simulink library "DAEMOT_Lib"  (R2019b)
settings: Solver=ode45  StartTime=0.0  StopTime=10.0  FixedStep=0.1  RelTol=1e-3
undefined symbols (not defined in the file or in its folder): Controller, CP, Ctrl, Ctrl_Fcn, Elec1, f, F2, Fluid, lag1, Mission, Moody, PropellerProp, rev_comms_sink
libraries: $bdroot x200, instrumentlib x21, simulink x5, dspsigops x2
(part 10 of 13)

== system DAEMOT_Lib/Support Functions/Real-Time Communication ==
  note: These blocks can be used to debug a controller that you want to run on hardware. With these blocks, the controller can be verified with a simulated plant. When transitioning to the hardware, simply replace these blocks with the non-debug version. At some point, it may be useful to combine the debug and non-debug versions into a single block. Maybe a task best saved for a rainy day :)
  note: We might be able to merge these two. I was never able to figure out if a combined block affected the output? However, the split format may be better for debugging purposes...
  LabVIEW_UDP : Subsystem  mask(LabView Measurements){n_in=[], n_out=[], config_loc=C:\Users\aksland2\BoxS\Box Sync\Research\Graduate Research\Models\UDP Communications Blocks\Matlab.json}
      mask prompts: n_in "Number of measurements from LabView"; n_out "Number of measurements to LabView"; config_loc "LabVIEW Config File Location (.json)"
      mask help: This block sends data to and from LabVIEW over UDP. The bus names are taken from a configuration file generated within LabVIEW. The update rate is hard-coded to 10 Hz.
      mask init:
      | h      = get_param(gcb,'handle');   % Get block handle
      | blk    = gcb;
      | hblock = get(h);     % Parse out handles structure
      | 
      | % Load .json file
      | fname = config_loc;
      | fid = fopen(fname);
      | raw = fread(fid,inf);
      | str = char(raw');
      | fclose(fid);
      | val = jsondecode(str);
      | 
      | % Retrieve data of interest
      | signals_in = val{1,1};
      | signals_out = val{2,1};
      | 
      | % Remove empty cells
      | signals_in  = signals_in(~cellfun(@isempty,signals_in));
      | signals_out = signals_out(~cellfun(@isempty,signals_out));
      | 
      | n_in  = length(signals_in);
      | n_out = length(signals_out);
      | 
      | % Set Demux and Bus Creator dimensions
      | set_param([blk,'/Demux'],'Outputs',num2str(n_in));
      | set_param([blk,'/Bus Creator'],'Inputs',num2str(n_in));
      | set_param([blk,'/UDP Receive/'],'DataSize',['[', num2str(n_in), ' 1]']);
      | 
      | % Get line handles
      | p = get_param([blk,'/Demux'],'PortHandles');
      | % l = get_param(p.Outport,'Line');
      | 
      | for i=1:n_in
      |     try
      |         % Draw lines
      |         add_line(blk,['Demux/',num2str(i)], ['Bus Creator/',num2str(i)],'AutoRouting','on')
      |     catch
      |         set_param(p.Outport(i),'Name',signals_in{i})
      |     end
      | end
      | 
      | delete_unconnected_lines(blk);
      | 
      | % Generate string of bus names to LabVIEW
      | out_str = '';
      | for i=1:n_out-1
      |     out_str = [out_str,[signals_out{i},',']];
      | end
      | out_str = [out_str,signals_out{n_out}];
      | 
      | set_param([blk,'/Bus Selector'],'OutputSignals',out_str);
      mask Display:
      | port_label('input',1,['Bus to LabVIEW - ',num2str(n_out),' signals'])
      | port_label('output',1,['Bus from LabVIEW - ',num2str(n_in),' signals'])
  UDP_Controller : Subsystem  Priority=2  mask{ctrl_fcn=[1*u(1)], conn=1, update_rate=.1, send_rate=Ctrl.dtSend, in_size=10, out_size=10, port_in=61177, loc_port_in=61176, port_out=61167, loc_port_out=61166}
      mask prompts: ctrl_fcn "Controller Function Name"; conn "Connection Number [1-10]"; update_rate "Controller Update Rate (s)"; send_rate "Send Rate [s]"; in_size "Controller Input Size"; out_size "Controller Output Size"; port_in "Input Port"; loc_port_in "Input Local Port"; port_out "Output Port"; loc_port_out "Output Local Port"
      mask help: Solves a controller with inputs/outputs sent over a UDP connection. The UDP Receive sample time is set to the controller update rate.
      mask init:
      | block = gcb;
      | 
      | port_in     = '61577';
      | loc_port_in = '61576';
      | 
      | port_out     = '61567';
      | loc_port_out = '61566';
      | 
      | port_in      = [port_in(1:2)     ,conn,port_in(4:5)];
      | loc_port_in  = [loc_port_in(1:2) ,conn,loc_port_in(4:5)];
      | port_out     = [port_out(1:2)    ,conn,port_out(4:5)];
      | loc_port_out = [loc_port_out(1:2),conn,loc_port_out(4:5)];
      | 
      | set_param(gcb,'port_in'     ,port_in);
      | set_param(gcb,'loc_port_in' ,loc_port_in);
      | set_param(gcb,'port_out'    ,port_out);
      | set_param(gcb,'loc_port_out',loc_port_out);
      | 
      | set_param([gcb,'/Controller/Controller'],'MATLABFcn',ctrl_fcn);
      | set_param([gcb,'/Controller/Controller'],'OutputDimensions',num2str(out_size));
      | set_param([gcb,'/Controller'],'SystemSampleTime',num2str(update_rate));
      | 
      | set_param([gcb,'/UDP Receive'],'Port',port_in);
      | set_param([gcb,'/UDP Receive'],'LocalPort',loc_port_in);
      | set_param([gcb,'/UDP Receive'],'SampleTime',num2str(update_rate));
      | set_param([gcb,'/UDP Receive'],'Timeout',num2str(update_rate+5));
      | set_param([gcb,'/UDP Receive'],'DataSize',['[', num2str(in_size), ' 1]']);
      | 
      | 
      | 
      | % set_param([gcb,'/From Controller'],'SystemSampleTime',num2str(update_rate));
      | set_param([gcb,'/From Controller/UDP Send'],'Port',port_out);
      | set_param([gcb,'/From Controller/UDP Send'],'LocalPort',loc_port_out);
      | set_param([gcb,'/From Controller'],'SystemSampleTime',num2str(update_rate));
      | 
      | set_param(bdroot,'FixedStep',num2str(update_rate))
      mask Display:
      | disp(['UDP Controller\n\nFunction: ',ctrl_fcn,'\n\nConnection: ',conn,'\n\nUpdate Rate (s): ',num2str(update_rate),'s\n\nInput Size: ',num2str(in_size),'\n\nOutput Size: ',num2str(out_size)])
      | 
      | % disp(['UDP Controller\n\nFunction: ',ctrl_fcn,'\n\nConnection: ',conn,'\n\nUpdate Rate (s): ',num2str(update_rate),'\n\nSend Rate (s): ',num2str(send_rate),'s\n\nInput Size: ',num2str(in_size),'\n\nOutput Size: ',num2str(out_size)])
  UDP_Controller_Debug : Subsystem  Priority=2  AncestorBlock=DAEMOT_Lib_2016a/Support Functions/UDP_Controller  mask{ctrl_fcn=Controller(u), conn=1, update_rate=.1, send_rate=.1, in_size=10, out_size=10, port_in=61177, loc_port_in=61176, port_out=61167, loc_port_out=61166}
      mask prompts: ctrl_fcn "Controller Function Name"; conn "Connection Number [1-10]"; update_rate "Controller Update Rate (s)"; send_rate "Send Rate [s]"; in_size "Controller Input Size"; out_size "Controller Output Size"; port_in "Input Port"; loc_port_in "Input Local Port"; port_out "Output Port"; loc_port_out "Output Local Port"
      mask help: Solves a controller with inputs/outputs sent over a UDP connection. The UDP Receive sample time is set to the controller update rate.
      mask init:
      | block = gcb;
      | 
      | port_in     = '61577';
      | loc_port_in = '61576';
      | 
      | port_out     = '61567';
      | loc_port_out = '61566';
      | 
      | port_in      = [port_in(1:2)     ,conn,port_in(4:5)];
      | loc_port_in  = [loc_port_in(1:2) ,conn,loc_port_in(4:5)];
      | port_out     = [port_out(1:2)    ,conn,port_out(4:5)];
      | loc_port_out = [loc_port_out(1:2),conn,loc_port_out(4:5)];
      | 
      | set_param(gcb,'port_in'     ,port_in);
      | set_param(gcb,'loc_port_in' ,loc_port_in);
      | set_param(gcb,'port_out'    ,port_out);
      | set_param(gcb,'loc_port_out',loc_port_out);
      | 
      | set_param([gcb,'/Controller'],'MATLABFcn',ctrl_fcn);
      | set_param([gcb,'/Controller'],'OutputDimensions',num2str(out_size));
      | 
      | set_param([gcb,'/UDP Receive'],'Port',port_in);
      | set_param([gcb,'/UDP Receive'],'LocalPort',loc_port_in);
      | set_param([gcb,'/UDP Receive'],'SampleTime',num2str(update_rate));
      | set_param([gcb,'/UDP Receive'],'Timeout',num2str(update_rate+5));
      | set_param([gcb,'/UDP Receive'],'DataSize',['[', num2str(in_size), ' 1]']);
      | 
      | 
      | 
      | % set_param([gcb,'/From Controller'],'SystemSampleTime',num2str(update_rate));
      | set_param([gcb,'/From Controller/UDP Send'],'Port',port_out);
      | set_param([gcb,'/From Controller/UDP Send'],'LocalPort',loc_port_out);
      | set_param([gcb,'/From Controller'],'SystemSampleTime',num2str(send_rate));
      | 
      | set_param(bdroot,'FixedStep',num2str(update_rate))
      mask Display: disp(['UDP Controller\n\nFunction: ',ctrl_fcn,'\n\nConnection: ',conn,'\n\nUpdate Rate (s): ',num2str(update_rate),'\n\nSend Rate (s): ',num2str(send_rate),'s\n\nInput Size: ',num2str(in_size),'\n\nOutput Size: ',num2str(out_size)])
  UDP_Controller_Recieve : Subsystem  mask(Send/Receive to UDP Controller){conn=1, update_rate=.1, rec_rate=.1, out_size=10, Initial=zeros(10,1), port_out=61166, loc_port_out=61167}
      mask prompts: conn "Connection Number [1-10]"; update_rate "Controller Update Rate (s)"; rec_rate "Recieve Rate [s]"; out_size "Controller Output Size"; Initial "Initial Output"; port_out "Output Port"; loc_port_out "Output Local Port"
      mask help: Sends and retrieves data from a controller over a UDP connection. Passes data over UDP at 10 Hz but applies a sample and hold at the update rate of the controller.
      mask init:
      | block = gcb;
      | 
      | % port_in     = '61576';
      | % loc_port_in = '61577';
      | 
      | port_out     = '61566';
      | loc_port_out = '61567';
      | 
      | % port_in      = [port_in(1:2)     ,conn,port_in(4:5)];
      | % loc_port_in  = [loc_port_in(1:2) ,conn,loc_port_in(4:5)];
      | port_out     = [port_out(1:2)    ,conn,port_out(4:5)];
      | loc_port_out = [loc_port_out(1:2),conn,loc_port_out(4:5)];
      | % 
      | % set_param(gcb,'port_in'     ,port_in);
      | % set_param(gcb,'loc_port_in' ,loc_port_in);
      | set_param(gcb,'port_out'    ,port_out);
      | set_param(gcb,'loc_port_out',loc_port_out);
      | % 
      | % set_param([gcb,'/To Controller/UDP Send'],'Port',port_in);
      | % set_param([gcb,'/To Controller/UDP Send'],'LocalPort',loc_port_in);
      | 
      | % test2 = ['[', num2str(out_size), ' 1]']
      | set_param([gcb,'/UDP Receive'],'Port',port_out);
      | set_param([gcb,'/UDP Receive'],'LocalPort',loc_port_out);
      | set_param([gcb,'/UDP Receive'],'DataSize',['[', num2str(out_size), ' 1]']);
      | set_param([gcb,'/UDP Receive'],'SampleTime',num2str(rec_rate));
      | 
      | set_param([gcb,'/Zero-Order Hold'],'SampleTime',num2str(update_rate));
      mask Display: disp(['Receive from UDP Controller\n\nConnection: ',conn,'\n\nUpdate Rate (s): ',num2str(update_rate),'\n\nReceive Rate (s): ',num2str(rec_rate),'\n\nOutput Size: ',num2str(out_size)])
  UDP_Controller_Recieve_Debug : Subsystem  Priority=3  AncestorBlock=DAEMOT_Lib_2016a/Support Functions/UDP_Controller_SR  mask(Send/Receive to UDP Controller){conn=1, update_rate=10, rec_rate=.1, out_size=10, Initial=zeros(10,1), port_out=61166, loc_port_out=61167}
      mask prompts: conn "Connection Number [1-10]"; update_rate "Controller Update Rate (s)"; rec_rate "Recieve Rate [s]"; out_size "Controller Output Size"; Initial "Initial Output"; port_out "Output Port"; loc_port_out "Output Local Port"
      mask help: Sends and retrieves data from a controller over a UDP connection. Passes data over UDP at 10 Hz but applies a sample and hold at the update rate of the controller.
      mask init:
      | block = gcb;
      | 
      | % port_in     = '61576';
      | % loc_port_in = '61577';
      | 
      | port_out     = '61566';
      | loc_port_out = '61567';
      | 
      | % port_in      = [port_in(1:2)     ,conn,port_in(4:5)];
      | % loc_port_in  = [loc_port_in(1:2) ,conn,loc_port_in(4:5)];
      | port_out     = [port_out(1:2)    ,conn,port_out(4:5)];
      | loc_port_out = [loc_port_out(1:2),conn,loc_port_out(4:5)];
      | % 
      | % set_param(gcb,'port_in'     ,port_in);
      | % set_param(gcb,'loc_port_in' ,loc_port_in);
      | set_param(gcb,'port_out'    ,port_out);
      | set_param(gcb,'loc_port_out',loc_port_out);
      | % 
      | % set_param([gcb,'/To Controller/UDP Send'],'Port',port_in);
      | % set_param([gcb,'/To Controller/UDP Send'],'LocalPort',loc_port_in);
      | 
      | % test2 = ['[', num2str(out_size), ' 1]']
      | set_param([gcb,'/UDP Receive'],'Port',port_out);
      | set_param([gcb,'/UDP Receive'],'LocalPort',loc_port_out);
      | set_param([gcb,'/UDP Receive'],'DataSize',['[', num2str(out_size), ' 1]']);
      | set_param([gcb,'/UDP Receive'],'SampleTime',num2str(rec_rate));
      mask Display: disp(['Receive from UDP Controller\n\nConnection: ',conn,'\n\nUpdate Rate (s): ',num2str(update_rate),'\n\nReceive Rate (s): ',num2str(rec_rate),'\n\nOutput Size: ',num2str(out_size)])
  UDP_Controller_Send : Subsystem  mask(Send/Receive to UDP Controller){conn=1, update_rate=.1, in_size=10, port_in=61176, loc_port_in=61177}
      mask prompts: conn "Connection Number [1-10]"; update_rate "Controller Update Rate (s)"; in_size "Controller Input Size"; port_in "Input Port"; loc_port_in "Input Local Port"
      mask help: Sends and retrieves data from a controller over a UDP connection. Passes data over UDP at 10 Hz but applies a sample and hold at the update rate of the controller.
      mask init:
      | block = gcb;
      | 
      | port_in     = '61576';
      | loc_port_in = '61577';
      | 
      | % port_out     = '61566';
      | % loc_port_out = '61567';
      | 
      | port_in      = [port_in(1:2)     ,conn,port_in(4:5)];
      | loc_port_in  = [loc_port_in(1:2) ,conn,loc_port_in(4:5)];
      | % port_out     = [port_out(1:2)    ,conn,port_out(4:5)];
      | % loc_port_out = [loc_port_out(1:2),conn,loc_port_out(4:5)];
      | 
      | set_param(gcb,'port_in'     ,port_in);
      | set_param(gcb,'loc_port_in' ,loc_port_in);
      | % set_param(gcb,'port_out'    ,port_out);
      | % set_param(gcb,'loc_port_out',loc_port_out);
      | 
      | set_param([gcb,'/To Controller/UDP Send'],'Port',port_in);
      | set_param([gcb,'/To Controller/UDP Send'],'LocalPort',loc_port_in);
      | set_param([gcb,'/To Controller'],'SystemSampleTime',num2str(update_rate));
      | 
      | % set_param([gcb,'/From Controller/MEASUREMENTS1/UDP Receive'],'Port',port_out);
      | % set_param([gcb,'/From Controller/MEASUREMENTS1/UDP Receive'],'LocalPort',loc_port_out);
      mask Display:
      | disp(['Send to UDP Controller\n\nConnection: ',conn,'\n\nUpdate Rate (s): ',num2str(update_rate),'s\n\nInput Size: ',num2str(in_size)])
      | % disp(['Send/Receive to UDP Controller\n\nConnection: ',conn,'\n\nUpdate Rate (s): ',num2str(update_rate),'s\n\nInput Size: ',num2str(in_size),'\n\nOutput Size: ',num2str(out_size)])
  UDP_Controller_Send_Debug : Subsystem  Priority=1  AncestorBlock=DAEMOT_Lib_2016a/Support Functions/UDP_Controller_SR  mask(Send/Receive to UDP Controller){conn=1, update_rate=.1, in_size=10, port_in=61176, loc_port_in=61177}
      mask prompts: conn "Connection Number [1-10]"; update_rate "Controller Update Rate (s)"; in_size "Controller Input Size"; port_in "Input Port"; loc_port_in "Input Local Port"
      mask help: Sends and retrieves data from a controller over a UDP connection. Passes data over UDP at 10 Hz but applies a sample and hold at the update rate of the controller.
      mask init: same as DAEMOT_Lib/Support Functions/Real-Time Communication/UDP_Controller_Send
      mask Display:
      | disp(['Send to UDP Controller\n\nConnection: ',conn,'\n\nUpdate Rate (s): ',num2str(update_rate),'s\n\nInput Size: ',num2str(in_size)])
      | % disp(['Send/Receive to UDP Controller\n\nConnection: ',conn,'\n\nUpdate Rate (s): ',num2str(update_rate),'s\n\nInput Size: ',num2str(in_size),'\n\nOutput Size: ',num2str(out_size)])

== system DAEMOT_Lib/Support Functions/Sink ==
  In1 : Inport
  tag scope: gdata_DAEMOT_LibSupportFunctionsSink=global
  wires:
  In1/1 -> [gdata_DAEMOT_LibSupportFunctionsSink]

== system DAEMOT_Lib/Support Functions/Source ==
  Out1 : Outport  VectorParamsAs1DForOutWhenUnconnected=off
  wires:
  [gdata_Thermal_System_BUSM2FSink2] -> Out1/1

== system DAEMOT_Lib/Support Functions/Unit Conversion  ==
  Signal_in : Inport
  conv_fcn : Fcn  Expr=(u(1)+459.67)/1.8-273.15
  Converted Signal Out : Outport  VectorParamsAs1DForOutWhenUnconnected=off
  wires:
  conv_fcn/1 -> Converted Signal Out/1
  Signal_in/1 -> conv_fcn/1

== system DAEMOT_Lib/Support Functions/Upper to Lower Edge Preview ==
  Trajectory : Inport
  Digital Clock : DigitalClock  SampleTime=dt_u
  Mission Preview1 : Subsystem  TreatAsAtomicUnit=on  SystemSampleTime=dt_l
  Scope : Scope
  Reference : Outport
  wires:
  Mission Preview1/1(References) -> Reference/1, Scope/1
  Trajectory/1 -> Mission Preview1/1(Trajectory)
  Digital Clock/1 -> Mission Preview1/2(Time)

== system DAEMOT_Lib/Support Functions/Upper to Lower Mission Preview ==
  Current State : Inport
  Trajectory : Inport  Port=2
  Bias1 : Bias  Bias=dt_l*linspace(0,(hor_l-1),hor_l)+dt_l
  Constant : Constant  Value=opts
  Constant1 : Constant  Value=dt_u*linspace(1,hor_u,hor_u)
  Constant2 : Constant  Value=ones(hor_u,1)  SampleTime=-1
  Constant4 : Constant  Value=dt_u  SampleTime=-1
  Digital Clock1 : DigitalClock  SampleTime=dt_l
  Lookup Table Dynamic : simulink/Lookup Tables/Lookup Table Dynamic  LookUpMeth=Interpolation-Use End Values  OutDataType=fixdt('double')  OutScaling=[]  OutputDataTypeScalingMode=Specify via dialog  OutDataTypeStr=fixdt('double')  DoSatur=off
      settings: SourceProductName=Simulink
  Math Function : Math  Operator=mod  SaturateOnIntegerOverflow=on
  Mux1 : Mux  Inputs=2
  Mux2 : Mux  Inputs=2
  Product : Product
  Selector : Selector  InputPortWidth=hor_u  IndexOptions=Index vector (dialog)  Indices=1  OutputSizes=1
  Switch : Switch  Criteria=u2 > Threshold
  Reference : Outport  VectorParamsAs1DForOutWhenUnconnected=off
  wires:
  Constant4/1 -> Math Function/2
  Digital Clock1/1 -> Math Function/1
  Constant/1 -> Switch/2
  Switch/1 -> Mux1/2
  Current State/1 -> Mux1/1
  Trajectory/1 -> Selector/1, Switch/3
  Mux1/1 -> Lookup Table Dynamic/3
  Mux2/1 -> Lookup Table Dynamic/2
  Constant1/1 -> Mux2/2
  Math Function/1 -> Bias1/1, Mux2/1
  Bias1/1 -> Lookup Table Dynamic/1
  Lookup Table Dynamic/1 -> Reference/1
  Product/1 -> Switch/1
  Selector/1 -> Product/2
  Constant2/1 -> Product/1

== system DAEMOT_Lib/Thermal/Air Volume ==
  In1 : Inport
  In2 : Inport  Port=2
  Q : Inport  Port=3
  Air_Volume : MATLAB Function  TreatAsAtomicUnit=on
  Bus Creator2 : BusCreator  Inputs=3
  Bus Selector1 : BusSelector  OutputSignals=Q_kW,Temp
  Constant : Constant  Value=P_init
  Constant1 : Constant  Value=T_init
  Data_Sink1 : $bdroot/Support Functions/Data_Sink
  Demux : Demux  Outputs=3
  Integrate : Integrator  InitialCondition=[T_init P_init M_init]  LimitOutput=on
  Sink1 : $bdroot/Support Functions/Sink
  Sink2 : $bdroot/Support Functions/Sink  Commented=on
  Source1 : $bdroot/Support Functions/Source
  Terminator : Terminator
  Terminator1 : Terminator
  b1 : BusCreator  Inputs=3
  gb1 : BusSelector  OutputSignals=mdot_kgps,T_C,P_kPa
  kW to W : Gain  Gain=1e3
  n-D Lookup Table1 : Lookup_n-D  BreakpointsForDimension1=Fluid.P  BreakpointsForDimension2=Fluid.T  BreakpointsForDimension3=[5, 7]  Table=Fluid.C_pt  ExtrapMethod=Clip  UseLastTableValue=on  RndMeth=Simplest  InputSameDT=on
  n-D Lookup Table2 : Lookup_n-D  BreakpointsForDimension1=Fluid.P  BreakpointsForDimension2=Fluid.T  BreakpointsForDimension3=[5, 7]  Table=Fluid.Rho_pt  ExtrapMethod=Clip  UseLastTableValue=on  RndMeth=Simplest  InputSameDT=on
  pout1 : From  Commented=on  GotoTag=T_tank
  Out1 : Outport  VectorParamsAs1DForOutWhenUnconnected=off
  wires:
  b1/1 -> Out1/1
  [Mdot_out] -> b1/1  "mdot_kgps"
  gb1/2 -> [T_in]  "<T_C>"
  [T_tank] -> b1/2  "T_C"
  gb1/1 -> [Mdot_in]  "<mdot_kgps>"
  In1/1 -> gb1/1
  [P_tank] -> b1/3  "P_kPa"
  gb1/3 -> Terminator/1  "<P_kPa>"
  [P_tank] -> Sink1/1
  Source1/1 -> [Mdot_out]
  In2/1 -> [T_amb]
  [Mdot_in] -> Air_Volume/2(Mdot_in)
  [Mdot_out] -> Air_Volume/3(Mdot_out)
  Air_Volume/1(x_dot) -> Integrate/1
  Integrate/1 -> Air_Volume/1(x), Demux/1
  Demux/1 -> [T_tank]
  Demux/2 -> [P_tank]
  Constant1/1 -> n-D Lookup Table2/2, n-D Lookup Table1/2
  Constant/1 -> n-D Lookup Table2/1, n-D Lookup Table1/1
  n-D Lookup Table1/1 -> Air_Volume/6(Cp)
  n-D Lookup Table2/1 -> Air_Volume/7(Rho)
  [T_in] -> Air_Volume/4(T_in)
  [T_amb] -> Air_Volume/5(T_amb)
  Bus Creator2/1 -> Data_Sink1/1
  [T_tank] -> Bus Creator2/1  "T"
  [P_tank] -> Bus Creator2/2  "P"
  [M_tank] -> Bus Creator2/3  "M"
  kW to W/1 -> Air_Volume/8(Q)
  Demux/3 -> [M_tank]
  pout1/1 -> Sink2/1
  Bus Selector1/2 -> Terminator1/1  "<Temp>"
  Bus Selector1/1 -> kW to W/1  "<Q_kW>"
  Q/1 -> Bus Selector1/1

== system DAEMOT_Lib/Thermal/Cold_Plate ==
  In1 : Inport
  Q : Inport  Port=2
  Bus Creator2 : BusCreator  Inputs=7
  Bus Selector : BusSelector  OutputSignals=Q_kW,Temp
  Cold_Plate : MATLAB Function  TreatAsAtomicUnit=on
  Constant2 : Constant  Value=Fluid.Bulk_Mod
  Demux : Demux  Outputs=3
  Integrate : Integrator  InitialCondition=[T_init P_init Tw_init]
  Mdot : MATLAB Function  TreatAsAtomicUnit=on
  Sink1 : $bdroot/Support Functions/Sink
  Sink2 : $bdroot/Support Functions/Sink
  Source1 : $bdroot/Support Functions/Source
  Terminator : Terminator
  Terminator2 : Terminator
  b1 : BusCreator  Inputs=3
  data_sink1 : $bdroot/Support Functions/Data_Sink
  gb1 : BusSelector  OutputSignals=mdot_kgps,T_C,P_kPa
  n-D Lookup Table1 : Lookup_n-D  BreakpointsForDimension1=Fluid.P  BreakpointsForDimension2=Fluid.T  BreakpointsForDimension3=[5, 7]  Table=Fluid.C_pt  ExtrapMethod=Clip  UseLastTableValue=on  RndMeth=Simplest  InputSameDT=on
  n-D Lookup Table2 : Lookup_n-D  BreakpointsForDimension1=Fluid.P  BreakpointsForDimension2=Fluid.T  BreakpointsForDimension3=[5, 7]  Table=Fluid.Rho_pt  ExtrapMethod=Clip  UseLastTableValue=on  RndMeth=Simplest  InputSameDT=on
  n-D Lookup Table8 : Lookup_n-D  BreakpointsForDimension1=Fluid.P  BreakpointsForDimension2=Fluid.T  BreakpointsForDimension3=[5, 7]  Table=Fluid.K_pt  ExtrapMethod=Clip  UseLastTableValue=on  RndMeth=Simplest  InputSameDT=on
  n-D Lookup Table9 : Lookup_n-D  BreakpointsForDimension1=Fluid.P  BreakpointsForDimension2=Fluid.T  BreakpointsForDimension3=[5, 7]  Table=Fluid.Mu_pt  ExtrapMethod=Clip  UseLastTableValue=on  RndMeth=Simplest  InputSameDT=on
  Out1 : Outport  VectorParamsAs1DForOutWhenUnconnected=off
  wires:
  b1/1 -> Out1/1
  [Mdot_down] -> b1/1  "mdot_kgps"
  gb1/2 -> [T_in]  "<T_C>"
  [T_out] -> b1/2  "T_C"
  gb1/1 -> Terminator2/1  "<mdot_kgps>"
  In1/1 -> gb1/1
  [P_out] -> b1/3  "P_kPa"
  gb1/3 -> [P_in]  "<P_kPa>"
  [Mdot] -> Sink1/1
  [Q_Load] -> Cold_Plate/2(Q_load)
  Source1/1 -> [Mdot_down]
  [T_in] -> Cold_Plate/6(T_in)
  Cold_Plate/1(x_dot) -> Integrate/1
  Bus Creator2/1 -> data_sink1/1
  [T_wall] -> Bus Creator2/4  "T_wall"
  [T_out] -> Bus Creator2/3  "T_out"
  [P_out] -> Bus Creator2/2  "P_out"
  [Q_Load] -> Bus Creator2/5  "Q_load"
  [Mdot] -> Bus Creator2/1  "Mdot"
  Cold_Plate/2(H) -> [H]  "HTC (W/m^2K)"
  [H] -> Bus Creator2/6  "HTC"
  n-D Lookup Table8/1 -> Cold_Plate/8(k)
  n-D Lookup Table9/1 -> Cold_Plate/7(mu)
  [T_out] -> n-D Lookup Table2/2, n-D Lookup Table9/2, n-D Lookup Table1/2, n-D Lookup Table8/2
  Integrate/1 -> Cold_Plate/1(x), Demux/1
  n-D Lookup Table1/1 -> Cold_Plate/9(Cp)
  Constant2/1 -> Cold_Plate/11(E_fluid)
  [Mdot_down] -> Cold_Plate/4(Mdot_down)
  [P_in] -> Cold_Plate/3(P_in)
  n-D Lookup Table2/1 -> Mdot/3(Rho), Cold_Plate/10(Rho)
  Mdot/1(Mdot) -> [Mdot], Cold_Plate/5(Mdot)
  [P_in] -> Mdot/1(P_in)
  [P_out] -> Mdot/2(P_out)
  Demux/2 -> [P_out]
  Demux/1 -> [T_out]
  Demux/3 -> [T_wall]
  [P_out] -> n-D Lookup Table2/1, n-D Lookup Table1/1, n-D Lookup Table8/1, n-D Lookup Table9/1
  Cold_Plate/3(Re) -> [Re]  "Re"
  [Re] -> Bus Creator2/7  "Re"
  Q/1 -> Bus Selector/1
  Bus Selector/1 -> [Q_Load]  "<Q_kW>"
  [T_wall] -> Sink2/1
  Bus Selector/2 -> Terminator/1  "<Temp>"

== system DAEMOT_Lib/Thermal/Flow Split_Junction ==
  In1 : Inport
  Bus Creator2 : BusCreator  Inputs=2
  Constant5 : Constant  Value=Fluid.Bulk_Mod
  Demux : Demux  Outputs=2
  Dynamic_Flow_Split_Junction : MATLAB Function  TreatAsAtomicUnit=on
  Integrator1 : Integrator  InitialCondition=[T_init P_init]
  Mux_In_1 : Mux  Inputs=1
  Mux_In_2 : Mux  Inputs=1
  Mux_In_3 : Mux  Inputs=1
  Selector1 : Selector  InputPortWidth=1  IndexOptions=Index vector (dialog)  Indices=[1 ]  OutputSizes=1
  Selector2 : Selector  InputPortWidth=1  IndexOptions=Index vector (dialog)  Indices=[1 ]  OutputSizes=1
  Sink1 : $bdroot/Support Functions/Sink
  Source1 : Subsystem
      mask init:
      | n_src = gcb;
      | n_src = str2num(n_src(end));
      | 
      | rev_comms_source(n_src);
      mask Display: text(0.25,0.5,'Source')
  b1 : BusCreator  Inputs=3
  data_sink1 : $bdroot/Support Functions/Data_Sink
  gb1 : BusSelector  OutputSignals=mdot_kgps,T_C,P_kPa
  gp1 : Terminator
  n-D Lookup Table2 : Lookup_n-D  BreakpointsForDimension1=Fluid.P  BreakpointsForDimension2=Fluid.T  BreakpointsForDimension3=[5, 7]  Table=Fluid.Rho_pt  ExtrapMethod=Clip  UseLastTableValue=on  RndMeth=Simplest  InputSameDT=on
  Out1 : Outport  VectorParamsAs1DForOutWhenUnconnected=off
  wires:
  b1/1 -> Out1/1
  [M_out1] -> b1/1  "mdot_kgps"
  gb1/2 -> [T_in1]  "<T_C>"
  [T] -> b1/2  "T_C"
  gb1/1 -> [M_in1]  "<mdot_kgps>"
  Source1/1(Out1) -> [M_out1]
  In1/1 -> gb1/1
  [P] -> b1/3  "P_kPa"
  gb1/3 -> gp1/1  "<P_kPa>"
  Mux_In_3/1 -> Selector2/1
  Mux_In_1/1 -> Selector1/1
  Mux_In_2/1 -> Dynamic_Flow_Split_Junction/3(Mdot_out)
  [M_in1] -> Mux_In_1/1
  [M_out1] -> Mux_In_2/1
  [T_in1] -> Mux_In_3/1
  [P] -> Sink1/1
  Dynamic_Flow_Split_Junction/1(x_dot) -> Integrator1/1
  Bus Creator2/1 -> data_sink1/1
  [T] -> Bus Creator2/1  "T_out"
  [P] -> Bus Creator2/2  "P"
  Integrator1/1 -> Demux/1, Dynamic_Flow_Split_Junction/1(x)
  Selector1/1 -> Dynamic_Flow_Split_Junction/2(Mdot_in)
  Constant5/1 -> Dynamic_Flow_Split_Junction/6(E_fluid)
  n-D Lookup Table2/1 -> Dynamic_Flow_Split_Junction/5(rho)
  [P] -> n-D Lookup Table2/1
  [T] -> n-D Lookup Table2/2
  Demux/1 -> [T]
  Demux/2 -> [P]
  Selector2/1 -> Dynamic_Flow_Split_Junction/4(T_in)

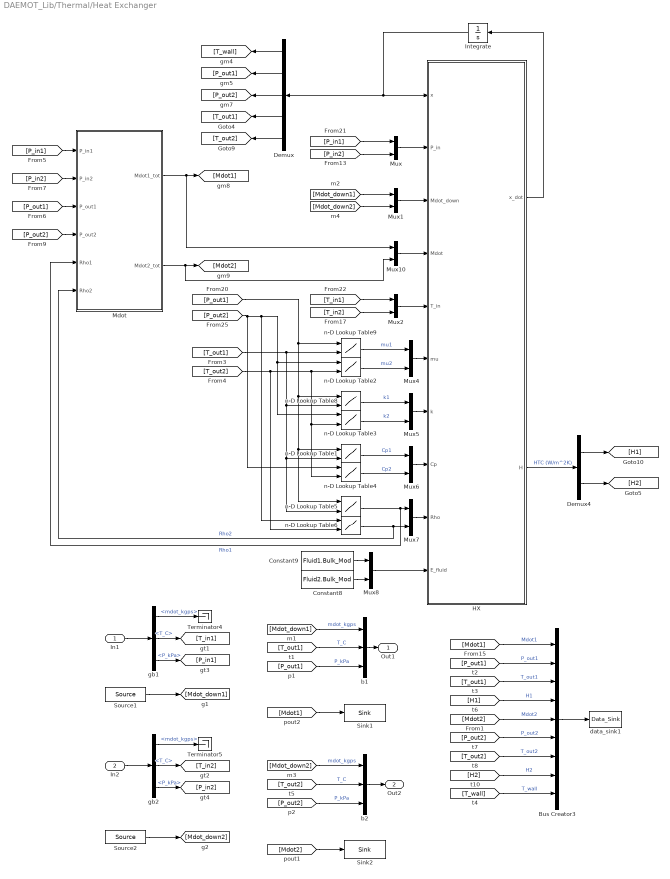
== system DAEMOT_Lib/Thermal/Heat Exchanger ==
  In1 : Inport
  In2 : Inport  Port=2
  Bus Creator3 : BusCreator  Inputs=9
  Constant8 : Constant  Value=Fluid2.Bulk_Mod
  Constant9 : Constant  Value=Fluid1.Bulk_Mod
  Demux : Demux  Outputs=5
  Demux4 : Demux  Outputs=2
  HX : MATLAB Function  TreatAsAtomicUnit=on
  Integrate : Integrator  InitialCondition=[Tw_init P1_init P2_init T1_init T2_init]
  Mdot : MATLAB Function  TreatAsAtomicUnit=on
  Mux{,1..2,4..8,10} (9 alike) : Mux  Inputs=2
  Sink1 : $bdroot/Support Functions/Sink
  Sink2 : $bdroot/Support Functions/Sink
  Source1 : $bdroot/Support Functions/Source
  Source2 : $bdroot/Support Functions/Source
  Terminator4 : Terminator
  Terminator5 : Terminator
  b1 : BusCreator  Inputs=3
  b2 : BusCreator  Inputs=3
  data_sink1 : $bdroot/Support Functions/Data_Sink
  gb1 : BusSelector  OutputSignals=mdot_kgps,T_C,P_kPa
  gb2 : BusSelector  OutputSignals=mdot_kgps,T_C,P_kPa
  n-D Lookup Table1 : Lookup_n-D  BreakpointsForDimension1=Fluid1.P  BreakpointsForDimension2=Fluid1.T  BreakpointsForDimension3=[5, 7]  Table=Fluid1.C_pt  ExtrapMethod=Clip  RndMeth=Simplest  InputSameDT=on
  n-D Lookup Table2 : Lookup_n-D  BreakpointsForDimension1=Fluid2.P  BreakpointsForDimension2=Fluid2.T  BreakpointsForDimension3=[5, 7]  Table=Fluid2.Mu_pt  ExtrapMethod=Clip  UseLastTableValue=on  RndMeth=Simplest  InputSameDT=on
  n-D Lookup Table3 : Lookup_n-D  BreakpointsForDimension1=Fluid2.P  BreakpointsForDimension2=Fluid2.T  BreakpointsForDimension3=[5, 7]  Table=Fluid2.K_pt  ExtrapMethod=Clip  UseLastTableValue=on  RndMeth=Simplest  InputSameDT=on
  n-D Lookup Table4 : Lookup_n-D  BreakpointsForDimension1=Fluid2.P  BreakpointsForDimension2=Fluid2.T  BreakpointsForDimension3=[5, 7]  Table=Fluid2.C_pt  ExtrapMethod=Clip  UseLastTableValue=on  RndMeth=Simplest  InputSameDT=on
  n-D Lookup Table5 : Lookup_n-D  BreakpointsForDimension1=Fluid1.P  BreakpointsForDimension2=Fluid1.T  BreakpointsForDimension3=[5, 7]  Table=Fluid1.Rho_pt  ExtrapMethod=Clip  UseLastTableValue=on  RndMeth=Simplest  InputSameDT=on
  n-D Lookup Table6 : Lookup_n-D  BreakpointsForDimension1=Fluid2.P  BreakpointsForDimension2=Fluid2.T  BreakpointsForDimension3=[5, 7]  Table=Fluid2.Rho_pt  ExtrapMethod=Clip  UseLastTableValue=on  RndMeth=Simplest  InputSameDT=on
  n-D Lookup Table8 : Lookup_n-D  BreakpointsForDimension1=Fluid1.P  BreakpointsForDimension2=Fluid1.T  BreakpointsForDimension3=[5, 7]  Table=Fluid1.K_pt  ExtrapMethod=Clip  UseLastTableValue=on  RndMeth=Simplest  InputSameDT=on
  n-D Lookup Table9 : Lookup_n-D  BreakpointsForDimension1=Fluid1.P  BreakpointsForDimension2=Fluid1.T  BreakpointsForDimension3=[5, 7]  Table=Fluid1.Mu_pt  ExtrapMethod=Clip  UseLastTableValue=on  RndMeth=Simplest  InputSameDT=on
  Out1 : Outport  VectorParamsAs1DForOutWhenUnconnected=off
  Out2 : Outport  Port=2  VectorParamsAs1DForOutWhenUnconnected=off
  wires:
  b1/1 -> Out1/1
  [Mdot_down1] -> b1/1  "mdot_kgps"
  gb1/2 -> [T_in1]  "<T_C>"
  [T_out1] -> b1/2  "T_C"
  gb1/1 -> Terminator4/1  "<mdot_kgps>"
  In1/1 -> gb1/1
  [P_out1] -> b1/3  "P_kPa"
  gb1/3 -> [P_in1]  "<P_kPa>"
  [Mdot1] -> Sink1/1
  [P_in1] -> Mux/1
  Source1/1 -> [Mdot_down1]
  [Mdot_down1] -> Mux1/1
  [T_in1] -> Mux2/1
  HX/1(x_dot) -> Integrate/1
  Integrate/1 -> Demux/1, HX/1(x)
  Demux/1 -> [T_wall]
  Demux/2 -> [P_out1]
  HX/2(H) -> Demux4/1  "HTC (W/m^2K)"
  n-D Lookup Table8/1 -> Mux5/1  "k1"
  n-D Lookup Table9/1 -> Mux4/1  "mu1"
  [T_out1] -> n-D Lookup Table9/2, n-D Lookup Table5/2, n-D Lookup Table1/2, n-D Lookup Table8/2
  [P_out1] -> n-D Lookup Table5/1, n-D Lookup Table1/1, n-D Lookup Table8/1, n-D Lookup Table9/1
  n-D Lookup Table1/1 -> Mux6/1  "Cp1"
  n-D Lookup Table5/1 -> Mdot/5(Rho1), Mux7/1  "Rho1"
  gb2/2 -> [T_in2]  "<T_C>"
  gb2/1 -> Terminator5/1  "<mdot_kgps>"
  In2/1 -> gb2/1
  gb2/3 -> [P_in2]  "<P_kPa>"
  Source2/1 -> [Mdot_down2]
  b2/1 -> Out2/1
  [Mdot_down2] -> b2/1  "mdot_kgps"
  [T_out2] -> b2/2  "T_C"
  [P_out2] -> b2/3  "P_kPa"
  [Mdot2] -> Sink2/1
  Mux/1 -> HX/2(P_in)
  [P_in2] -> Mux/2
  Mux1/1 -> HX/3(Mdot_down)
  [Mdot_down2] -> Mux1/2
  Mux2/1 -> HX/5(T_in)
  [T_in2] -> Mux2/2
  Mux4/1 -> HX/6(mu)
  n-D Lookup Table2/1 -> Mux4/2  "mu2"
  [P_out2] -> n-D Lookup Table4/1, n-D Lookup Table6/1, n-D Lookup Table3/1, n-D Lookup Table2/1
  [T_out2] -> n-D Lookup Table3/2, n-D Lookup Table4/2, n-D Lookup Table2/2, n-D Lookup Table6/2
  Mux5/1 -> HX/7(k)
  n-D Lookup Table3/1 -> Mux5/2  "k2"
  Mux6/1 -> HX/8(Cp)
  n-D Lookup Table4/1 -> Mux6/2  "Cp2"
  Mux7/1 -> HX/9(Rho)
  Mux8/1 -> HX/10(E_fluid)
  Demux4/1 -> [H1]
  Demux4/2 -> [H2]
  Demux/3 -> [P_out2]
  Constant9/1 -> Mux8/1
  Constant8/1 -> Mux8/2
  [H2] -> Bus Creator3/8  "H2"
  [T_out2] -> Bus Creator3/7  "T_out2"
  [P_out2] -> Bus Creator3/6  "P_out2"
  [Mdot2] -> Bus Creator3/5  "Mdot2"
  [H1] -> Bus Creator3/4  "H1"
  [T_out1] -> Bus Creator3/3  "T_out1"
  [T_wall] -> Bus Creator3/9  "T_wall"
  [P_out1] -> Bus Creator3/2  "P_out1"
  [Mdot1] -> Bus Creator3/1  "Mdot1"
  Bus Creator3/1 -> data_sink1/1
  [P_in1] -> Mdot/1(P_in1)
  n-D Lookup Table6/1 -> Mdot/6(Rho2), Mux7/2  "Rho2"
  [P_in2] -> Mdot/2(P_in2)
  [P_out2] -> Mdot/4(P_out2)
  Demux/4 -> [T_out1]
  Demux/5 -> [T_out2]
  Mdot/1(Mdot1_tot) -> Mux10/1, [Mdot1]
  Mux10/1 -> HX/4(Mdot)
  Mdot/2(Mdot2_tot) -> Mux10/2, [Mdot2]
  [P_out1] -> Mdot/3(P_out1)

== system DAEMOT_Lib/Thermal/Heat_Sink_Edge ==
  In1 : Inport
  Bus Creator : BusCreator  Inputs=1
  Bus Creator1 : BusCreator  Inputs=2
  Bus Selector : BusSelector  OutputSignals=Q_kW,Temp
  Data_Sink : $bdroot/Support Functions/Data_Sink
  Sink1 : $bdroot/Support Functions/Sink
  Source1 : $bdroot/Support Functions/Source
  Terminator : Terminator
  Thermal : MATLAB Function  TreatAsAtomicUnit=on
  Out1 : Outport  VectorParamsAs1DForOutWhenUnconnected=off
  wires:
  Thermal/1(Q) -> [Q]
  [T_source] -> Thermal/1(T_source)
  [Q] -> Bus Creator1/1  "Q_kW"
  Source1/1 -> [T_sink]
  Bus Selector/1 -> Terminator/1  "<Q_kW>"
  Bus Creator/1 -> Data_Sink/1
  [Q] -> Bus Creator/1  "Heat Flow"
  [T_sink] -> Thermal/2(T_sink)
  [Q] -> Sink1/1
  Bus Creator1/1 -> Out1/1
  In1/1 -> Bus Selector/1  "Therm"
  [T_sink] -> Bus Creator1/2  "Temp"
  Bus Selector/2 -> [T_source]  "<Temp>"

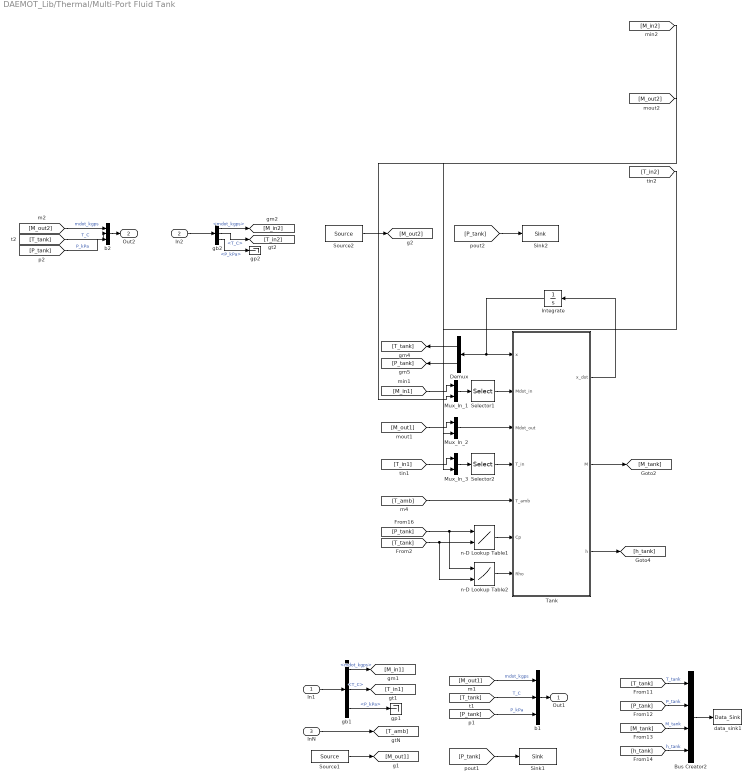
== system DAEMOT_Lib/Thermal/Multi-Port Fluid Tank ==
  In1 : Inport
  In2 : Inport  Port=2
  InN : Inport  Port=3
  Bus Creator2 : BusCreator  Inputs=4
  Demux : Demux  Outputs=2
  Integrate : Integrator  InitialCondition=[T_init P_init]
  Mux_In_1 : Mux  Inputs=2
  Mux_In_2 : Mux  Inputs=2
  Mux_In_3 : Mux  Inputs=2
  Selector1 : Selector  InputPortWidth=2  IndexOptions=Index vector (dialog)  Indices=[1 2 ]  OutputSizes=1
  Selector2 : Selector  InputPortWidth=2  IndexOptions=Index vector (dialog)  Indices=[1 2 ]  OutputSizes=1
  Sink1 : $bdroot/Support Functions/Sink
  Sink2 : $bdroot/Support Functions/Sink
  Source1 : $bdroot/Support Functions/Source
  Source2 : $bdroot/Support Functions/Source
  Tank : MATLAB Function  TreatAsAtomicUnit=on
  b1 : BusCreator  Inputs=3
  b2 : BusCreator  Inputs=3
  data_sink1 : $bdroot/Support Functions/Data_Sink
  gb1 : BusSelector  OutputSignals=mdot_kgps,T_C,P_kPa
  gb2 : BusSelector  OutputSignals=mdot_kgps,T_C,P_kPa
  gp1 : Terminator
  gp2 : Terminator
  n-D Lookup Table1 : Lookup_n-D  BreakpointsForDimension1=Fluid.P  BreakpointsForDimension2=Fluid.T  BreakpointsForDimension3=[5, 7]  Table=Fluid.C_pt  ExtrapMethod=Clip  UseLastTableValue=on  RndMeth=Simplest  InputSameDT=on
  n-D Lookup Table2 : Lookup_n-D  BreakpointsForDimension1=Fluid.P  BreakpointsForDimension2=Fluid.T  BreakpointsForDimension3=[5, 7]  Table=Fluid.Rho_pt  ExtrapMethod=Clip  UseLastTableValue=on  RndMeth=Simplest  InputSameDT=on
  Out1 : Outport  VectorParamsAs1DForOutWhenUnconnected=off
  Out2 : Outport  Port=2  VectorParamsAs1DForOutWhenUnconnected=off
  wires:
  Selector2/1 -> Tank/4(T_in)
  Selector1/1 -> Tank/2(Mdot_in)
  [T_in1] -> Mux_In_3/1
  [M_out1] -> Mux_In_2/1
  [M_in1] -> Mux_In_1/1
  Mux_In_2/1 -> Tank/3(Mdot_out)
  Mux_In_1/1 -> Selector1/1
  Mux_In_3/1 -> Selector2/1
  [M_tank] -> Bus Creator2/3  "M_tank"
  [h_tank] -> Bus Creator2/4  "h_tank"
  [P_tank] -> Bus Creator2/2  "P_tank"
  [T_tank] -> Bus Creator2/1  "T_tank"
  Bus Creator2/1 -> data_sink1/1
  [T_amb] -> Tank/5(T_amb)
  n-D Lookup Table2/1 -> Tank/7(Rho)
  Tank/2(M) -> [M_tank]
  n-D Lookup Table1/1 -> Tank/6(Cp)
  [P_tank] -> n-D Lookup Table1/1, n-D Lookup Table2/1
  [T_tank] -> n-D Lookup Table1/2, n-D Lookup Table2/2
  Tank/3(h) -> [h_tank]
  Demux/2 -> [P_tank]
  Demux/1 -> [T_tank]
  Integrate/1 -> Tank/1(x), Demux/1
  Tank/1(x_dot) -> Integrate/1
  InN/1 -> [T_amb]
  Source1/1 -> [M_out1]
  [P_tank] -> Sink1/1
  gb1/3 -> gp1/1  "<P_kPa>"
  [P_tank] -> b1/3  "P_kPa"
  In1/1 -> gb1/1
  gb1/1 -> [M_in1]  "<mdot_kgps>"
  [T_tank] -> b1/2  "T_C"
  gb1/2 -> [T_in1]  "<T_C>"
  [M_out1] -> b1/1  "mdot_kgps"
  b1/1 -> Out1/1
  In2/1 -> gb2/1
  gb2/1 -> [M_in2]  "<mdot_kgps>"
  gb2/2 -> [T_in2]  "<T_C>"
  gb2/3 -> gp2/1  "<P_kPa>"
  [P_tank] -> Sink2/1
  [M_in2] -> Mux_In_1/2
  [T_in2] -> Mux_In_3/2
  [M_out2] -> b2/1  "mdot_kgps"
  [T_tank] -> b2/2  "T_C"
  [P_tank] -> b2/3  "P_kPa"
  b2/1 -> Out2/1
  Source2/1 -> [M_out2]
  [M_out2] -> Mux_In_2/2

== system DAEMOT_Lib/Thermal/PCM Module ==
  Cooling In : Inport
  Bus Creator : BusCreator  Inputs=6
  Bus Creator1 : BusCreator  Inputs=2
  Bus Selector1 : BusSelector  OutputSignals=Q_kW,Temp
  Data_Sink : $bdroot/Support Functions/Data_Sink
  Demux : Demux  Outputs=3
  Gain : Gain  Gain=1/depth
  Gain2 : Gain  Gain=-1/1000
  Gain3 : Gain  Gain=1/1000
  Gain4 : Gain  Gain=1000
  Gain5 : Gain  Gain=-1/1000
  Integrator : Integrator  InitialCondition=T_1_0
  Integrator Limited : Integrator  InitialCondition=V_L_0*depth  LimitOutput=on  UpperSaturationLimit=depth  LowerSaturationLimit=1e-5*depth
  Phase Change Material : MATLAB Function  TreatAsAtomicUnit=on
  Props : Subsystem
  Sink2 : $bdroot/Support Functions/Sink
  Source1 : $bdroot/Support Functions/Source
  Terminator : Terminator
  Cooling Out : Outport  VectorParamsAs1DForOutWhenUnconnected=off
  wires:
  [state] -> Bus Creator/6  "State"
  [T_2] -> Sink2/1
  Gain4/1 -> [Q_out]
  [X] -> Gain/1
  Phase Change Material/4(state) -> [state]
  Demux/3 -> [T_base]
  Demux/2 -> [T_2]
  Demux/1 -> [T_1]
  Gain5/1 -> Bus Creator1/1  "Q_kW"
  Props/1(props) -> Phase Change Material/5(props)
  [Q_out] -> Phase Change Material/1(Q_out)
  Integrator/1 -> Demux/1, Phase Change Material/4(T)
  [Q_out] -> Gain3/1  "Q_out"
  [Q_in] -> Gain2/1  "Q_in"
  [T_1] -> Bus Creator/3  "Inner Surface Temp"
  [T_2] -> Bus Creator/4  "Outer Surface Temp"
  Bus Selector1/1 -> Gain4/1  "<Q_kW>"
  [X] -> Phase Change Material/3(X)
  [T_base] -> Bus Creator1/2  "Temp"
  [T_i] -> Phase Change Material/2(T_i)
  Source1/1 -> [T_i]
  [Q_in] -> Gain5/1
  Bus Creator1/1 -> Cooling Out/1
  Bus Creator/1 -> Data_Sink/1
  Gain3/1 -> Bus Creator/2  "Q_out"
  Gain2/1 -> Bus Creator/1  "Q_in"
  Phase Change Material/3(Q_in) -> [Q_in]
  Gain/1 -> Bus Creator/5  "Liquid Fraction"
  Integrator Limited/1 -> [X]
  Phase Change Material/2(X_dot) -> Integrator Limited/1
  Phase Change Material/1(T_dot) -> Integrator/1
  Bus Selector1/2 -> Terminator/1  "<Temp>"
  Cooling In/1 -> Bus Selector1/1

== system DAEMOT_Lib/Thermal/Peristaltic_Pump ==
  note: Or maybe Pamb?
  note: Don't need any of this info
  note: Need to get Pressure 4 maybe? Or maybe use Pin?
  note: Don't need any value from upstream component -
      | unsure if this is needed
  note: Need to send calculated mass flow rate to upstream component
  In1 : Inport
  In2 : Inport  Port=2
  Bus Creator2 : BusCreator  Inputs=1
  Constant3 : Constant  Value=H_k
  MATLAB Function : MATLAB Function  TreatAsAtomicUnit=on
  Sink1 : $bdroot/Support Functions/Sink
  Source1 : $bdroot/Support Functions/Source
  Terminator : Terminator
  Terminator3 : Terminator
  b2 : BusCreator  Inputs=3
  data_sink1 : $bdroot/Support Functions/Data_Sink
  gb2 : BusSelector  OutputSignals=mdot_kgps,T_C,P_kPa
  Out1 : Outport  VectorParamsAs1DForOutWhenUnconnected=off
  Out2 : Outport  Port=2  VectorParamsAs1DForOutWhenUnconnected=off
  wires:
  [P_in] -> MATLAB Function/1(P)
  [Speed_in] -> MATLAB Function/2(w)
  MATLAB Function/1(mdot) -> [Mdot]
  [Mdot] -> Sink1/1
  Source1/1 -> Terminator/1
  In2/1 -> [Speed_in]
  gb2/3 -> [P_in]  "<P_kPa>"
  In1/1 -> gb2/1
  gb2/1 -> Terminator3/1  "<mdot_kgps>"
  gb2/2 -> [T_in]  "<T_C>"
  [P_out] -> b2/3  "P_kPa"
  [T_out] -> b2/2  "T_C"
  [Mdot] -> b2/1  "mdot_kgps"
  b2/1 -> Out1/1
  [P_in] -> [P_out]
  [T_in] -> [T_out]
  [Mdot] -> Bus Creator2/1  "Mdot"
  [Mdot] -> Out2/1
  Constant3/1 -> MATLAB Function/3(H_k)
  Bus Creator2/1 -> data_sink1/1

== system DAEMOT_Lib/Thermal/Pipe_P_to_M ==
  In1 : Inport
  In2 : Inport  Port=2
  Bus Creator2 : BusCreator  Inputs=3
  Constant2 : Constant  Value=Fluid.Bulk_Mod
  Demux : Demux  Outputs=2
  Integrate : Integrator  InitialCondition=[T_init P_init]
  Mdot : MATLAB Function  TreatAsAtomicUnit=on
  Pipe_P_to_M : MATLAB Function  TreatAsAtomicUnit=on
  Sink1 : $bdroot/Support Functions/Sink
  Source1 : $bdroot/Support Functions/Source
  Terminator1 : Terminator
  Terminator3 : Terminator
  b2 : BusCreator  Inputs=3
  data_sink1 : $bdroot/Support Functions/Data_Sink
  gb2 : BusSelector  OutputSignals=mdot_kgps,T_C,P_kPa
  n-D Lookup Table2 : Lookup_n-D  BreakpointsForDimension1=Fluid.P  BreakpointsForDimension2=Fluid.T  BreakpointsForDimension3=[5, 7]  Table=Fluid.Rho_pt  ExtrapMethod=Clip  UseLastTableValue=on  RndMeth=Simplest  InputSameDT=on
  Out1 : Outport  VectorParamsAs1DForOutWhenUnconnected=off
  wires:
  Bus Creator2/1 -> data_sink1/1
  [T_out] -> Bus Creator2/1  "T_out"
  [T_amb] -> Terminator1/1
  [T_out] -> n-D Lookup Table2/2
  [P_out] -> n-D Lookup Table2/1
  n-D Lookup Table2/1 -> Pipe_P_to_M/5(Rho), Mdot/3(Rho)
  [Mdot] -> Bus Creator2/2  "Mdot"
  [P_out] -> Bus Creator2/3  "P_out"
  Pipe_P_to_M/1(x_dot) -> Integrate/1
  Integrate/1 -> Pipe_P_to_M/1(x), Demux/1
  b2/1 -> Out1/1
  [Mdot_down] -> b2/1  "mdot_kgps"
  gb2/2 -> [T_in]  "<T_C>"
  [T_out] -> b2/2  "T_C"
  gb2/1 -> Terminator3/1  "<mdot_kgps>"
  In1/1 -> gb2/1
  [P_out] -> b2/3  "P_kPa"
  gb2/3 -> [P_in]  "<P_kPa>"
  [Mdot] -> Sink1/1
  Source1/1 -> [Mdot_down]
  In2/1 -> [T_amb]
  [Mdot_down] -> Pipe_P_to_M/3(Mdot_down)
  Constant2/1 -> Pipe_P_to_M/6(E_fluid)
  [T_in] -> Pipe_P_to_M/2(T_in)
  [P_in] -> Mdot/1(P_in)
  [P_out] -> Mdot/2(P_out)
  Mdot/1(Mdot) -> Pipe_P_to_M/4(Mdot), [Mdot]
  Demux/2 -> [P_out]
  Demux/1 -> [T_out]

== system DAEMOT_Lib/Thermal/Pipe_P_to_P ==
  In1 : Inport
  In2 : Inport  Port=2
  Bus Creator2 : BusCreator  Inputs=2
  Integrate1 : Integrator  InitialCondition=T_init
  Mdot : MATLAB Function  TreatAsAtomicUnit=on
  Pipe_P_to_M : MATLAB Function  TreatAsAtomicUnit=on
  Sink1 : $bdroot/Support Functions/Sink
  Source1 : $bdroot/Support Functions/Source
  Terminator1 : Terminator
  Terminator2 : Terminator
  b1 : BusCreator  Inputs=3
  data_sink1 : $bdroot/Support Functions/Data_Sink
  gb1 : BusSelector  OutputSignals=mdot_kgps,T_C,P_kPa
  n-D Lookup Table1 : Lookup_n-D  BreakpointsForDimension1=Fluid.P  BreakpointsForDimension2=Fluid.T  BreakpointsForDimension3=[5, 7]  Table=Fluid.Rho_pt  ExtrapMethod=Clip  UseLastTableValue=on  RndMeth=Simplest  InputSameDT=on
  Out1 : Outport  VectorParamsAs1DForOutWhenUnconnected=off
  wires:
  b1/1 -> Out1/1
  [Mdot] -> b1/1  "mdot_kgps"
  gb1/2 -> [T_in]  "<T_C>"
  [T_out] -> b1/2  "T_C"
  gb1/1 -> Terminator2/1  "<mdot_kgps>"
  In1/1 -> gb1/1
  [P_out] -> b1/3  "P_kPa"
  gb1/3 -> [P_in]  "<P_kPa>"
  [Mdot] -> Sink1/1
  Source1/1 -> [P_out]
  In2/1 -> [T_amb]
  Bus Creator2/1 -> data_sink1/1
  [T_out] -> Bus Creator2/1  "T_out"
  [T_amb] -> Terminator1/1
  [Mdot] -> Bus Creator2/2  "Mdot"
  Pipe_P_to_M/1(x_dot) -> Integrate1/1
  Integrate1/1 -> Pipe_P_to_M/1(x), [T_out]
  [T_in] -> Pipe_P_to_M/2(T_in)
  [T_out] -> n-D Lookup Table1/2
  [P_out] -> n-D Lookup Table1/1
  n-D Lookup Table1/1 -> Mdot/3(Rho), Pipe_P_to_M/4(Rho)
  [P_in] -> Mdot/1(P_in)
  [P_out] -> Mdot/2(P_out)
  Mdot/1(Mdot) -> [Mdot], Pipe_P_to_M/3(Mdot)

== system DAEMOT_Lib/Thermal/Pump ==
  In1 : Inport
  In2 : Inport  Port=2
  Bus Creator2 : BusCreator  Inputs=4
  Constant1 : Constant  Value=Fluid.Bulk_Mod
  Constant2 : Constant  Value=A
  Constant3 : Constant  Value=H_k
  Constant4 : Constant  Value=Rho_pump
  Constant5 : Constant  Value=Eta_k
  Demux : Demux  Outputs=2
  Integrate : Integrator  InitialCondition=[T_init P_init]
  Pump : MATLAB Function  TreatAsAtomicUnit=on
  Sink1 : $bdroot/Support Functions/Sink
  Source1 : $bdroot/Support Functions/Source
  Terminator1 : Terminator
  b1 : BusCreator  Inputs=3
  data_sink1 : $bdroot/Support Functions/Data_Sink
  gb1 : BusSelector  OutputSignals=mdot_kgps,T_C,P_kPa
  n-D Lookup Table6 : Lookup_n-D  BreakpointsForDimension1=Fluid.P  BreakpointsForDimension2=Fluid.T  BreakpointsForDimension3=[5, 7]  Table=Fluid.Rho_pt  ExtrapMethod=Clip  UseLastTableValue=on  RndMeth=Simplest  InputSameDT=on
  Out1 : Outport  VectorParamsAs1DForOutWhenUnconnected=off
  wires:
  b1/1 -> Out1/1
  [Mdot_down] -> b1/1  "mdot_kgps"
  gb1/2 -> [T_in]  "<T_C>"
  [T_out] -> b1/2  "T_C"
  gb1/1 -> Terminator1/1  "<mdot_kgps>"
  In1/1 -> gb1/1
  [P_out] -> b1/3  "P_kPa"
  gb1/3 -> [P_in]  "<P_kPa>"
  [Mdot] -> Sink1/1
  Source1/1 -> [Mdot_down]
  In2/1 -> [PWM]
  [PWM] -> Pump/5(PWM)
  Pump/3(Power) -> [Power]
  Bus Creator2/1 -> data_sink1/1
  [T_out] -> Bus Creator2/1  "T_out"
  [Mdot] -> Bus Creator2/2  "Mdot"
  [Power] -> Bus Creator2/4  "Power"
  [P_in] -> Pump/2(P_in)
  [Mdot_down] -> Pump/4(Mdot_down)
  Integrate/1 -> Pump/1(x), Demux/1
  Pump/1(x_dot) -> Integrate/1
  Constant1/1 -> Pump/6(E_fluid)
  n-D Lookup Table6/1 -> Pump/7(Rho)
  [P_out] -> n-D Lookup Table6/1
  [T_out] -> n-D Lookup Table6/2
  [T_in] -> Pump/3(T_in)
  [P_out] -> Bus Creator2/3  "P_out"
  Pump/2(Mdot) -> [Mdot]
  Demux/2 -> [P_out]
  Demux/1 -> [T_out]
  Constant2/1 -> Pump/8(A)
  Constant3/1 -> Pump/9(H_k)
  Constant4/1 -> Pump/10(Rho_pump)
  Constant5/1 -> Pump/11(Eta_k)

== system DAEMOT_Lib/Thermal/Specify_Mass_Flow_Rate ==
  In1 : Inport
  In2 : Inport  Port=2
  Bus Creator2 : BusCreator  Inputs=2
  Data_Sink : $bdroot/Support Functions/Data_Sink
  Sink1 : $bdroot/Support Functions/Sink
  Source1 : $bdroot/Support Functions/Source
  Terminator2 : Terminator
  b1 : BusCreator  Inputs=3
  gb1 : BusSelector  OutputSignals=mdot_kgps,T_C,P_kPa
  Out1 : Outport  VectorParamsAs1DForOutWhenUnconnected=off
  wires:
  In2/1 -> [Mdot]
  [Mdot] -> b1/1  "mdot_kgps"
  [T_in] -> Bus Creator2/1  "T_out"
  [T_in] -> b1/2  "T_C"
  Bus Creator2/1 -> Data_Sink/1
  [P_out] -> b1/3  "P_kPa"
  gb1/3 -> [P_in]  "<P_kPa>"
  [Mdot] -> Bus Creator2/2  "Mdot"
  In1/1 -> gb1/1
  [Mdot] -> Sink1/1
  Source1/1 -> [P_out]
  gb1/2 -> [T_in]  "<T_C>"
  b1/1 -> Out1/1
  gb1/1 -> Terminator2/1  "<mdot_kgps>"

== system DAEMOT_Lib/Thermal/Valve_P_to_M ==
  In1 : Inport
  In2 : Inport  Port=2
  Bus Creator2 : BusCreator  Inputs=3
  Constant2 : Constant  Value=Fluid.Bulk_Mod
  Demux : Demux  Outputs=2
  Integrate : Integrator  InitialCondition=[T_init P_init]
  Mdot : MATLAB Function  TreatAsAtomicUnit=on
  Pipe_P_to_M : MATLAB Function  TreatAsAtomicUnit=on
  Product : Product
  Saturation : Saturate  UpperLimit=1  LowerLimit=0
  Sink1 : $bdroot/Support Functions/Sink
  Source1 : $bdroot/Support Functions/Source
  Terminator3 : Terminator
  b2 : BusCreator  Inputs=3
  data_sink1 : $bdroot/Support Functions/Data_Sink
  gb2 : BusSelector  OutputSignals=mdot_kgps,T_C,P_kPa
  n-D Lookup Table2 : Lookup_n-D  BreakpointsForDimension1=Fluid.P  BreakpointsForDimension2=Fluid.T  BreakpointsForDimension3=[5, 7]  Table=Fluid.Rho_pt  ExtrapMethod=Clip  UseLastTableValue=on  RndMeth=Simplest  InputSameDT=on
  Out1 : Outport  VectorParamsAs1DForOutWhenUnconnected=off
  wires:
  Bus Creator2/1 -> data_sink1/1
  [T_out] -> Bus Creator2/1  "T_out"
  [T_out] -> n-D Lookup Table2/2
  [P_out] -> n-D Lookup Table2/1
  n-D Lookup Table2/1 -> Pipe_P_to_M/5(Rho), Mdot/3(Rho)
  [Mdot] -> Bus Creator2/2  "Mdot"
  [P_out] -> Bus Creator2/3  "P_out"
  Pipe_P_to_M/1(x_dot) -> Integrate/1
  Integrate/1 -> Pipe_P_to_M/1(x), Demux/1
  b2/1 -> Out1/1
  [Mdot_down] -> b2/1  "mdot_kgps"
  gb2/2 -> [T_in]  "<T_C>"
  [T_out] -> b2/2  "T_C"
  gb2/1 -> Terminator3/1  "<mdot_kgps>"
  In1/1 -> gb2/1
  [P_out] -> b2/3  "P_kPa"
  gb2/3 -> [P_in]  "<P_kPa>"
  [Mdot] -> Sink1/1
  Source1/1 -> [Mdot_down]
  In2/1 -> Saturation/1
  [Mdot_down] -> Pipe_P_to_M/3(Mdot_down)
  Constant2/1 -> Pipe_P_to_M/6(E_fluid)
  [T_in] -> Pipe_P_to_M/2(T_in)
  [P_in] -> Mdot/1(P_in)
  [P_out] -> Mdot/2(P_out)
  Demux/2 -> [P_out]
  Demux/1 -> [T_out]
  Product/1 -> [Mdot], Pipe_P_to_M/4(Mdot)
  Mdot/1(Mdot) -> Product/1
  [On_off] -> Product/2
  Saturation/1 -> [On_off]

== system DAEMOT_Lib/Thermal/Valve_P_to_P ==
  In1 : Inport
  In2 : Inport  Port=2
  Bus Creator2 : BusCreator  Inputs=2
  Integrate1 : Integrator  InitialCondition=T_init
  Mdot : MATLAB Function  TreatAsAtomicUnit=on
  Pipe_P_to_M : MATLAB Function  TreatAsAtomicUnit=on
  Product : Product
  Saturation : Saturate  UpperLimit=1  LowerLimit=0
  Sink1 : $bdroot/Support Functions/Sink
  Source1 : $bdroot/Support Functions/Source
  Terminator2 : Terminator
  b1 : BusCreator  Inputs=3
  data_sink1 : $bdroot/Support Functions/Data_Sink
  gb1 : BusSelector  OutputSignals=mdot_kgps,T_C,P_kPa
  n-D Lookup Table1 : Lookup_n-D  BreakpointsForDimension1=Fluid.P  BreakpointsForDimension2=Fluid.T  BreakpointsForDimension3=[5, 7]  Table=Fluid.Rho_pt  ExtrapMethod=Clip  UseLastTableValue=on  RndMeth=Simplest  InputSameDT=on
  Out1 : Outport  VectorParamsAs1DForOutWhenUnconnected=off
  wires:
  b1/1 -> Out1/1
  [Mdot] -> b1/1  "mdot_kgps"
  gb1/2 -> [T_in]  "<T_C>"
  [T_out] -> b1/2  "T_C"
  gb1/1 -> Terminator2/1  "<mdot_kgps>"
  In1/1 -> gb1/1
  [P_out] -> b1/3  "P_kPa"
  gb1/3 -> [P_in]  "<P_kPa>"
  [Mdot] -> Sink1/1
  Source1/1 -> [P_out]
  In2/1 -> Saturation/1
  Bus Creator2/1 -> data_sink1/1
  [T_out] -> Bus Creator2/1  "T_out"
  [Mdot] -> Bus Creator2/2  "Mdot"
  Pipe_P_to_M/1(x_dot) -> Integrate1/1
  Integrate1/1 -> Pipe_P_to_M/1(x), [T_out]
  [T_in] -> Pipe_P_to_M/2(T_in)
  [T_out] -> n-D Lookup Table1/2
  [P_out] -> n-D Lookup Table1/1
  n-D Lookup Table1/1 -> Mdot/3(Rho), Pipe_P_to_M/4(Rho)
  [P_in] -> Mdot/1(P_in)
  [P_out] -> Mdot/2(P_out)
  Product/1 -> [Mdot], Pipe_P_to_M/3(Mdot)
  Mdot/1(Mdot) -> Product/1
  [On_off] -> Product/2
  Saturation/1 -> [On_off]

== system DAEMOT_Lib/Electrical/Air Vehicle/Data_Sink ==
  " " : Inport
  tag scope: gdata_ElectricalAirVehicleData_Sink=global
  wires:
  " "/1 -> [gdata_ElectricalAirVehicleData_Sink]

== system DAEMOT_Lib/Electrical/Air Vehicle/Sink1 ==
  In1 : Inport
  tag scope: gdata_DAEMOT_LibElectricalAirVehicleSink1=global
  wires:
  In1/1 -> [gdata_DAEMOT_LibElectricalAirVehicleSink1]

== system DAEMOT_Lib/Electrical/Battery/Data_Sink ==
  " " : Inport
  tag scope: gdata_ElectricalBatteryData_Sink=global
  wires:
  " "/1 -> [gdata_ElectricalBatteryData_Sink]
